simulink model "transfer_function_signal_processing_example"  (R2021a)
settings: Solver=ode23t  StartTime=0.0  StopTime=0.25  RelTol=1e-3  AbsTol=1e-3
model workspace (MAT data in the model file):
  C = 3.4629e-05
  R = 228.5176
  Vo = [0 0.0001 0.0002 0.0003 0.0004 0.0005 0.0006 0.0007 0.0008 0.0009 0.001 0.0011 ... (5002 elements, 2501x2)]
libraries: fl_lib x7, nesl_utility x4, ee_lib x1
(part 1 of 2)
settings Model: OrderedModelArguments=off  Creator=Highlander  LastModifiedBy=Highlander
settings SolverCC: AutoScaleAbsTol=off  AlgebraicLoopSolver=TrustRegion
settings DebuggingCC: SymbolicDimsDataTypeCodeGenerationDiagnostic=none  SFMachineParentedDataDiag=warning
settings SFSimCC: CustomCodeUndefinedFunction=UseInterfaceOnly
settings SimscapeCC: SimscapeLogType=all  SimscapeLogSimulationStatistics=on  SimscapeLogDataHistory=10000

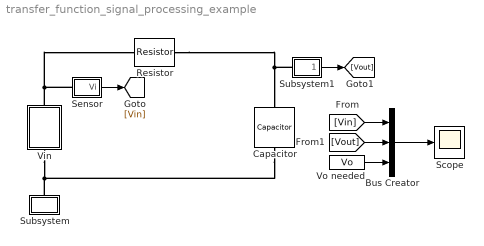
== system transfer_function_signal_processing_example ==
  Bus Creator : BusCreator  Inputs=3
  Capacitor : fl_lib/Electrical/Electrical Elements/Capacitor  c=C F  r=1e-6 Ohm  g=0 1/Ohm  i_specify=off  i_priority=None  i=0 A  i_nominal_specify=off  i_nominal_unit=A  i_nominal_value=1  v_specify=off  v_priority=High  v=0.2597 V  v_nominal_specify=off  v_nominal_unit=V  v_nominal_value=1  vc_specify=on  vc_priority=High  vc=0.904038236303809 V  vc_nominal_specify=off  vc_nominal_unit=V  vc_nominal_value=1
  Resistor : ee_lib/Passive/Resistor  R=R Ohm  R_tol=5  enable_R_tol=0  tol_distribution=1  nSigma=4  enable_operating_limits=0  operating_limit_action=2  max_working_voltage=100 V  power_rating=1 W  enable_faults=0  fault_action=1  R_faulted=inf Ohm  enable_temporal_fault=0  t_fault=1 s  enable_behavioral_fault=0  max_permissible_current=1 A  t_fail_on_current=1 s  noise_mode=0  sample_time=1e-3 s  repeatability=1  auto_seed=3499211588  user_seed=0  Tdevice=25 degC  alpha=3.93e-3 1/K  Tmeas=25 degC  thermal_mass=100 J/K  power_derating_T1=70 degC  power_derating_T2=155 degC  operating_temperature_range_vec=[-50, 150] degC  temperature_specify=off  temperature_priority=High  temperature=298.15 K  temperature_nominal_specify=off  temperature_nominal_unit=K  temperature_nominal_value=1
  Scope : Scope
  Sensor : Subsystem
      mask Display: disp("S")
  Subsystem : Subsystem
      mask Display: disp("gnd")
  Subsystem1 : Subsystem
      mask Display: disp("S")
  Vin : Subsystem
      mask Display: disp("Vin")
  Vo needed : FromWorkspace  VariableName=Vo
  wires:
  Bus Creator/1 -> Scope/1
  Vo needed/1 -> Bus Creator/3
  [Vin] -> Bus Creator/1
  Sensor/1(Vi) -> [Vin]
  Subsystem1/1(Vo estimated) -> [Vout]
  [Vout] -> Bus Creator/2
  connections:
  Resistor/RConn1 -- Subsystem1/LConn1 -- Capacitor/LConn1
  Sensor/LConn1 -- Resistor/LConn1 -- Vin/LConn1
  Subsystem/LConn1 -- Capacitor/RConn1 -- Vin/RConn1
